simulink model "shema_R2021a"  (R2021a)
settings: Solver=VariableStepAuto  StartTime=0.0  StopTime=30  RelTol=1e-5
undefined symbols (not defined in the file): b, dx0, F_0, k, m, t_F, x0
settings Model: Creator=Borna  LastModifiedBy=borna

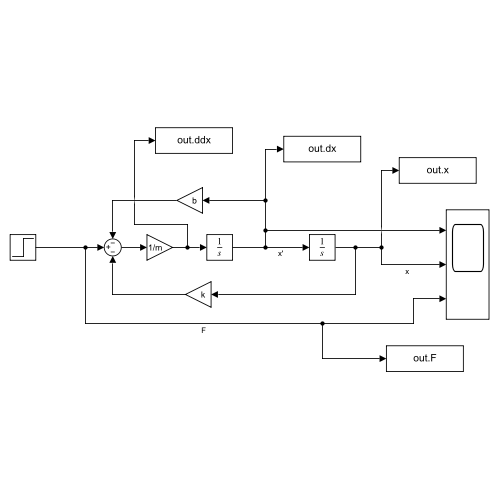
[thumbnail: Simulink's stored preview of the top-level diagram]
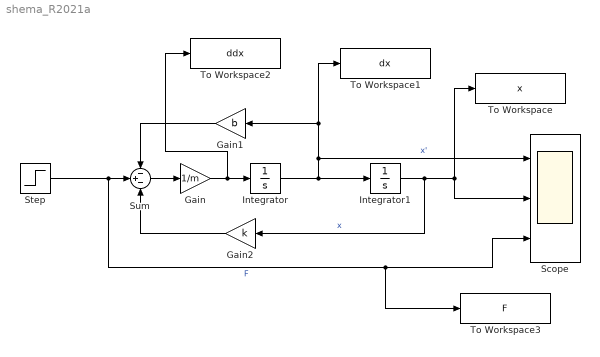
== system shema_R2021a ==
  Gain : Gain  Gain=1/m
  Gain1 : Gain  Gain=b
  Gain2 : Gain  Gain=k
  Integrator : Integrator  InitialCondition=dx0
  Integrator1 : Integrator  InitialCondition=x0
  Scope : Scope  NumInputPorts=3
  Step : Step  Time=t_F  After=F_0  SampleTime=0
  Sum : Sum  Inputs=-+-
  To Workspace : ToWorkspace  VariableName=x  SampleTime=-1
  To Workspace1 : ToWorkspace  VariableName=dx  SampleTime=-1
  To Workspace2 : ToWorkspace  VariableName=ddx  SampleTime=-1
  To Workspace3 : ToWorkspace  VariableName=F  SampleTime=-1
  wires:
  Integrator/1 -> To Workspace1/1, Gain1/1, Scope/1, Integrator1/1  "x'"
  Sum/1 -> Gain/1
  Gain/1 -> To Workspace2/1, Integrator/1
  Integrator1/1 -> To Workspace/1, Scope/2, Gain2/1  "x"
  Gain1/1 -> Sum/1
  Gain2/1 -> Sum/3
  Step/1 -> To Workspace3/1, Scope/3, Sum/2  "F"
